simulink model "ass6"  (R2022a)
settings: Solver=VariableStepAuto  StartTime=0.0  StopTime=10.0  RelTol=1e-3
values from neighbouring files (symbols this model uses):
  dDZ = 0.1    [initlab1sim.m]
  DZPOS = 0    [initlab1sim.m]
  TL = + 1.3    (= 1.3)    [initlab1sim.m]
  TU = - 1.0    (= -1)    [initlab1sim.m]
undefined symbols (not defined in the file or in its folder): SimDen, SimNum
settings Model: Creator=30416  LastModifiedBy=30416

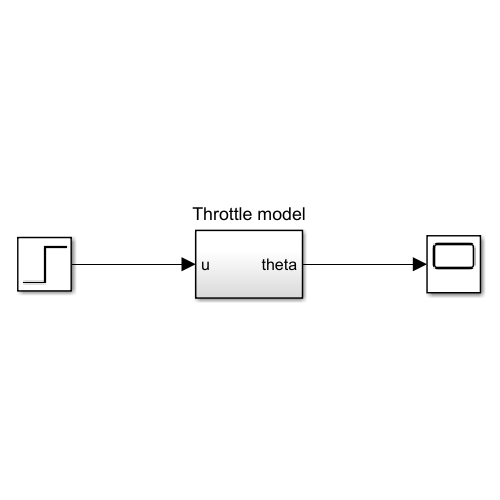
[thumbnail: Simulink's stored preview of the top-level diagram]
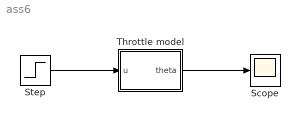
== system ass6 ==
  Scope : Scope
  Step : Step  After=10  SampleTime=0
  Throttle model : Subsystem
  wires:
  Step/1 -> Throttle model/1(u)
  Throttle model/1(theta) -> Scope/1

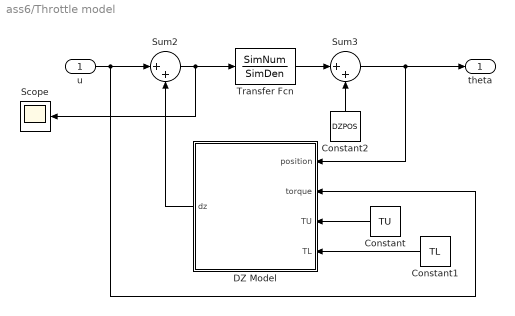
== system ass6/Throttle model ==
  u : Inport
  Constant : Constant  Value=TU
  Constant1 : Constant  Value=TL
  Constant2 : Constant  Value=DZPOS
  DZ Model : Subsystem
  Scope : Scope
  Sum2 : Sum  Inputs=|++  InputSameDT=on  SaturateOnIntegerOverflow=on  OutDataTypeStr=Inherit: Same as first input
  Sum3 : Sum  Inputs=|++  InputSameDT=on  SaturateOnIntegerOverflow=on  OutDataTypeStr=Inherit: Same as first input
  Transfer Fcn : TransferFcn  Numerator=SimNum  Denominator=SimDen
  theta : Outport
  wires:
  Sum3/1 -> DZ Model/1(position), theta/1
  Constant2/1 -> Sum3/2
  Transfer Fcn/1 -> Sum3/1
  u/1 -> DZ Model/2(torque), Sum2/1
  Constant/1 -> DZ Model/3(TU)
  Constant1/1 -> DZ Model/4(TL)
  Sum2/1 -> Transfer Fcn/1, Scope/1
  DZ Model/1(dz) -> Sum2/2

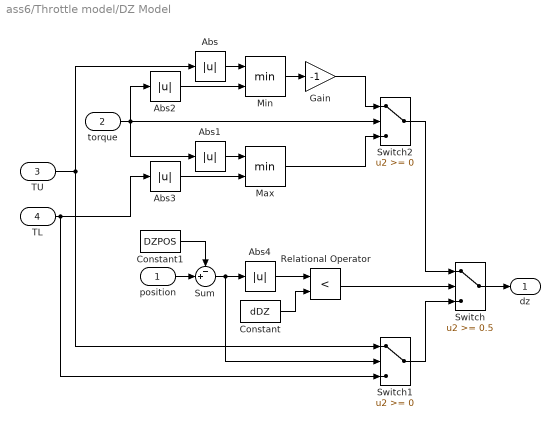
== system ass6/Throttle model/DZ Model ==
  position : Inport
  torque : Inport  Port=2
  TU : Inport  Port=3
  TL : Inport  Port=4
  Abs{,1..4} (5 alike) : Abs
  Constant : Constant  Value=dDZ
  Constant1 : Constant  Value=DZPOS
  Gain : Gain  Gain=-1  SaturateOnIntegerOverflow=on  OutDataTypeStr=Inherit: Same as input  ParamDataTypeStr=Inherit: Same as input
  Max : MinMax  Inputs=2  InputSameDT=on  SaturateOnIntegerOverflow=on
  Min : MinMax  Inputs=2  InputSameDT=on  SaturateOnIntegerOverflow=on
  Relational Operator : RelationalOperator  Operator=<
  Sum : Sum  Inputs=-+|  InputSameDT=on  SaturateOnIntegerOverflow=on  OutDataTypeStr=Inherit: Same as first input
  Switch : Switch  Threshold=0.5
  Switch1 : Switch
  Switch2 : Switch
  dz : Outport  InitialOutput=0
  wires:
  Abs4/1 -> Relational Operator/1
  Relational Operator/1 -> Switch/2
  Max/1 -> Switch2/3
  TL/1 -> Switch1/3, Abs3/1
  torque/1 -> Switch2/2, Abs1/1, Abs2/1
  TU/1 -> Switch1/1, Abs/1
  Abs/1 -> Min/1
  Abs1/1 -> Max/1
  Min/1 -> Gain/1
  Gain/1 -> Switch2/1
  Abs2/1 -> Min/2
  Abs3/1 -> Max/2
  Switch2/1 -> Switch/1
  Switch1/1 -> Switch/3
  Switch/1 -> dz/1
  Constant/1 -> Relational Operator/2
  position/1 -> Sum/2
  Constant1/1 -> Sum/1
  Sum/1 -> Abs4/1, Switch1/2
